simulink model "diff_mobile_model_2"  (R2015b)
settings: Solver=ode5  StartTime=0.0  StopTime=inf  FixedStep=0.01  RelTol=1e-3
values from neighbouring files (symbols this model uses):
  B = 0.1    [param.m]
  I = 0.8    [param.m]
  K = 1    [param.m]
  l = 0.2    [param.m]
  M = 20    [param.m]
  ppr = 1024*5    (= 5120)    [param.m]
  r = 0.065    [param.m]
  T = 0.01    [param.m]
libraries: simulink x2, slctrlblks x1
settings Model: Creator=root  LastModifiedBy=root

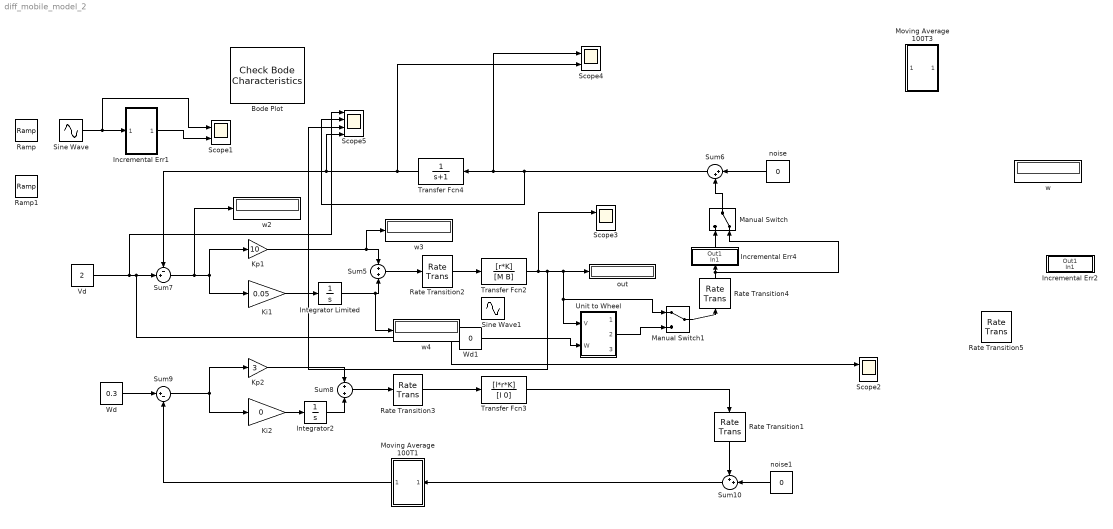
== system diff_mobile_model_2 ==
  Bode Plot : slctrlblks/Model Verification/Check Bode  Characteristics  InstantiateOnLoad=on  SaveOperatingPoints=off  LinearizationIOs={'/Sum7', 1, 'in', 'on', '';'/Transfer Fcn4', 1, 'out', 'on', ''}  LinearizeAt=SnapshotTimes  SnapshotTimes=[0]  TriggerType=rising  SampleTime=0.0001  RateConversionMethod=zoh  PreWarpFreq=10  UseExactDelayModel=off  UseFullBlockNameLabels=off  UseBusSignalLabels=off  enabled=on  stopWhenAssertionFail=off  export=off  ViewDlgPos=[66 1 767 793]  OpenViewOnLoad=on  LaunchViewOnOpen=on  FrequencyUnits=rad/s  MagnitudeUnits=dB  PhaseUnits=deg  TimeUnits=seconds  EnableUpperBound=off  UpperBoundFrequencies=[]  UpperBoundMagnitudes=[]  EnableLowerBound=off  LowerBoundFrequencies=[]  LowerBoundMagnitudes=[]
      settings: SaveToWorkspace=on
  Incremental Err1 : Subsystem
  Incremental Err2 : Subsystem
  Incremental Err4 : Subsystem
  Integrator Limited : Integrator  LimitOutput=on  UpperSaturationLimit=1000  LowerSaturationLimit=-1000
  Integrator2 : Integrator
  Ki1 : Gain  Gain=0.05
  Ki2 : Gain  Gain=0
  Kp1 : Gain  Gain=10
  Kp2 : Gain  Gain=3
  Manual Switch : ManualSwitch  CurrentSetting=0
  Manual Switch1 : ManualSwitch
  Moving Average 100T1 : Subsystem
  Moving Average 100T3 : Subsystem
  Ramp : simulink/Sources/Ramp  slope=1  start=0  X0=0
  Ramp1 : simulink/Sources/Ramp  slope=1  start=0  X0=0
  Rate Transition{1..5} (5 alike) : RateTransition  OutPortSampleTime=control_ts
  Scope{1..4} (4 alike) : Scope  NumInputPorts=2
  Scope5 : Scope  NumInputPorts=4
  Sine Wave : Sin  SampleTime=0
  Sine Wave1 : Sin  SampleTime=0
  Sum10 : Sum  Inputs=++|
  Sum5 : Sum  Inputs=+|+
  Sum6 : Sum  Inputs=|++
  Sum7 : Sum  Inputs=-+|
  Sum8 : Sum  Inputs=+|+
  Sum9 : Sum  Inputs=|+-
  Transfer Fcn2 : TransferFcn  Numerator=[r*K]  Denominator=[M B]
  Transfer Fcn3 : TransferFcn  Numerator=[l*r*K]  Denominator=[I 0]
  Transfer Fcn4 : TransferFcn  Denominator=[1 1]
  Unit to Wheel : Subsystem
  Vd : Constant  Value=2
  Wd : Constant  Value=0.3
  Wd1 : Constant  Value=0
  noise : Constant  Value=0
  noise1 : Constant  Value=0
  out : Display
  w{,2..4} (4 alike) : Display
  wires:
  noise/1 -> Sum6/1
  Kp1/1 -> w3/1, Sum5/1
  Ki1/1 -> Integrator Limited/1
  Sum5/1 -> Rate Transition2/1
  Sum7/1 -> w2/1, Ki1/1, Kp1/1
  Vd/1 -> Scope5/1, Scope2/1, Sum7/2
  Ki2/1 -> Integrator2/1
  Kp2/1 -> Sum8/1
  Integrator2/1 -> Sum8/2
  Sum8/1 -> Rate Transition3/1
  Sum9/1 -> Kp2/1, Ki2/1
  Wd/1 -> Sum9/1
  Transfer Fcn3/1 -> Rate Transition1/1
  noise1/1 -> Sum10/2
  Sum10/1 -> Moving Average 100T1/1(In1)
  Moving Average 100T1/1(Out1) -> Sum9/2
  Sine Wave/1 -> Scope1/1, Incremental Err1/1(In1)
  Incremental Err1/1(Out1) -> Scope1/2
  Rate Transition2/1 -> Transfer Fcn2/1
  Rate Transition1/1 -> Sum10/1
  Rate Transition3/1 -> Transfer Fcn3/1
  Rate Transition4/1 -> Manual Switch/2, Incremental Err4/1(In1)
  Wd1/1 -> Unit to Wheel/2(W)
  Transfer Fcn2/1 -> Scope3/1, Scope5/3, Manual Switch1/1, Unit to Wheel/1(V), out/1
  Manual Switch/1 -> Sum6/2
  Sum6/1 -> Scope5/2, Transfer Fcn4/1, Scope4/1
  Integrator Limited/1 -> w4/1, Sum5/2
  Transfer Fcn4/1 -> Scope4/2, Scope5/4, Sum7/1
  Incremental Err4/1(Out1) -> Manual Switch/1
  Manual Switch1/1 -> Rate Transition4/1
  Unit to Wheel/2(V_enc2) -> Manual Switch1/2

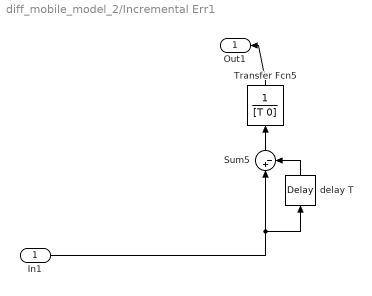
== system diff_mobile_model_2/Incremental Err1 ==
  In1 : Inport
  Sum5 : Sum  Inputs=|+-
  Transfer Fcn5 : TransferFcn  Denominator=[T 0]
  delay T : TransportDelay  DelayTime=T
  Out1 : Outport
  wires:
  Transfer Fcn5/1 -> Out1/1
  delay T/1 -> Sum5/2
  In1/1 -> Sum5/1, delay T/1
  Sum5/1 -> Transfer Fcn5/1

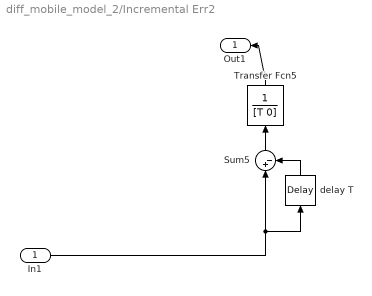
== system diff_mobile_model_2/Incremental Err2 ==
  In1 : Inport
  Sum5 : Sum  Inputs=|+-
  Transfer Fcn5 : TransferFcn  Denominator=[T 0]
  delay T : TransportDelay  DelayTime=T
  Out1 : Outport
  wires:
  Transfer Fcn5/1 -> Out1/1
  delay T/1 -> Sum5/2
  In1/1 -> Sum5/1, delay T/1
  Sum5/1 -> Transfer Fcn5/1

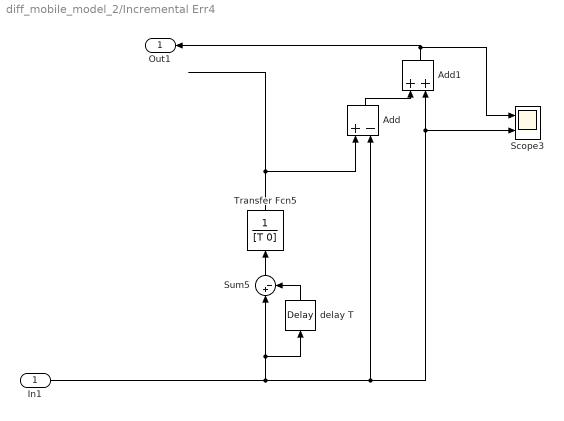
== system diff_mobile_model_2/Incremental Err4 ==
  In1 : Inport
  Add : Sum  Inputs=+-
  Add1 : Sum
  Scope3 : Scope  NumInputPorts=2
  Sum5 : Sum  Inputs=|+-
  Transfer Fcn5 : TransferFcn  Denominator=[T 0]
  delay T : TransportDelay  DelayTime=T
  Out1 : Outport
  wires:
  Transfer Fcn5/1 -> Add/1
  delay T/1 -> Sum5/2
  In1/1 -> Scope3/2, Add1/2, Add/2, Sum5/1, delay T/1
  Sum5/1 -> Transfer Fcn5/1
  Add/1 -> Add1/1
  Add1/1 -> Scope3/1, Out1/1

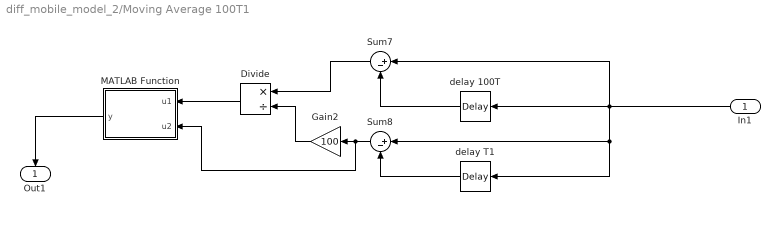
== system diff_mobile_model_2/Moving Average 100T1 ==
  In1 : Inport
  Divide : Product  Inputs=*/
  Gain2 : Gain  Gain=100
  MATLAB Function : MATLAB Function  TreatAsAtomicUnit=on
  Sum7 : Sum  Inputs=|+-
  Sum8 : Sum  Inputs=|+-
  delay 100T : TransportDelay  DelayTime=100
  delay T1 : TransportDelay  DelayTime=T
  Out1 : Outport
  wires:
  Divide/1 -> MATLAB Function/1(u1)
  Sum8/1 -> Gain2/1, MATLAB Function/2(u2)
  delay 100T/1 -> Sum7/2
  delay T1/1 -> Sum8/2
  In1/1 -> delay 100T/1, delay T1/1, Sum8/1, Sum7/1
  MATLAB Function/1(y) -> Out1/1
  Gain2/1 -> Divide/2
  Sum7/1 -> Divide/1

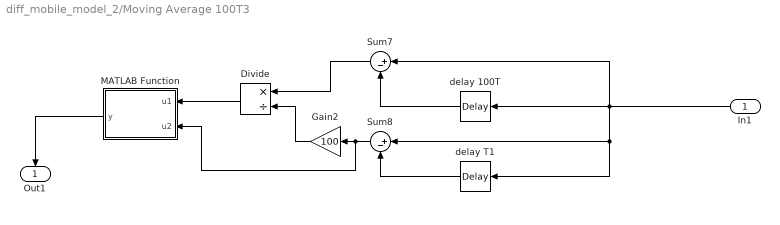
== system diff_mobile_model_2/Moving Average 100T3 ==
  In1 : Inport
  Divide : Product  Inputs=*/
  Gain2 : Gain  Gain=100
  MATLAB Function : MATLAB Function  TreatAsAtomicUnit=on
  Sum7 : Sum  Inputs=|+-
  Sum8 : Sum  Inputs=|+-
  delay 100T : TransportDelay  DelayTime=100
  delay T1 : TransportDelay  DelayTime=T
  Out1 : Outport
  wires:
  Sum7/1 -> Divide/1
  Gain2/1 -> Divide/2
  MATLAB Function/1(y) -> Out1/1
  In1/1 -> Sum7/1, Sum8/1, delay T1/1, delay 100T/1
  delay T1/1 -> Sum8/2
  delay 100T/1 -> Sum7/2
  Sum8/1 -> MATLAB Function/2(u2), Gain2/1
  Divide/1 -> MATLAB Function/1(u1)

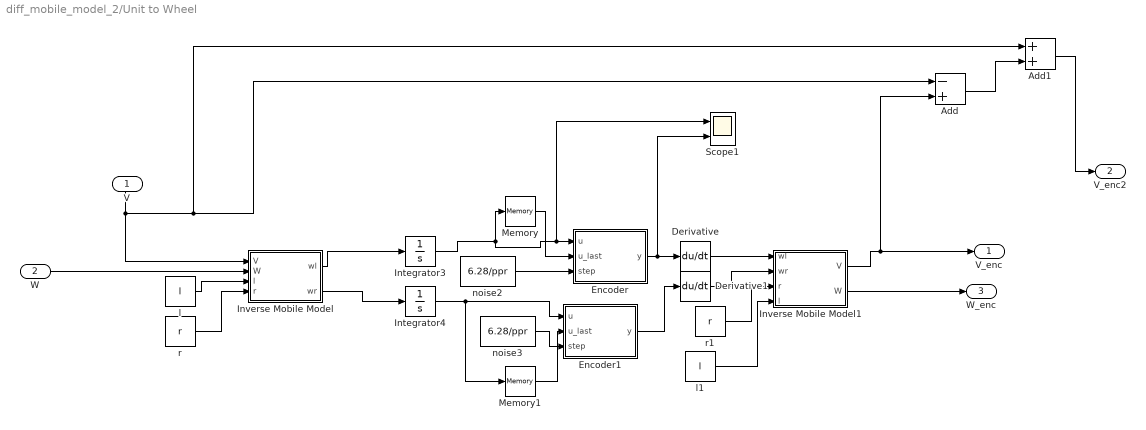
== system diff_mobile_model_2/Unit to Wheel ==
  V : Inport
  W : Inport  Port=2
  Add : Sum  Inputs=-+
  Add1 : Sum
  Derivative : Derivative
  Derivative1 : Derivative
  Encoder : MATLAB Function  TreatAsAtomicUnit=on
  Encoder1 : MATLAB Function  TreatAsAtomicUnit=on
  Integrator3 : Integrator
  Integrator4 : Integrator
  Inverse Mobile Model : MATLAB Function  TreatAsAtomicUnit=on
  Inverse Mobile Model1 : MATLAB Function  TreatAsAtomicUnit=on
  Memory : Memory
  Memory1 : Memory
  Scope1 : Scope  NumInputPorts=2
  l : Constant  Value=l
  l1 : Constant  Value=l
  noise2 : Constant  Value=6.28/ppr
  noise3 : Constant  Value=6.28/ppr
  r : Constant  Value=r
  r1 : Constant  Value=r
  V_enc : Outport
  V_enc2 : Outport  Port=2
  W_enc : Outport  Port=3
  wires:
  Inverse Mobile Model1/1(V) -> Add/2, V_enc/1
  Integrator4/1 -> Memory1/1, Encoder1/1(u)
  Integrator3/1 -> Memory/1, Scope1/1, Encoder/1(u)
  l/1 -> Inverse Mobile Model/3(l)
  Inverse Mobile Model1/2(W) -> W_enc/1
  Inverse Mobile Model/2(wr) -> Integrator4/1
  noise2/1 -> Encoder/3(step)
  W/1 -> Inverse Mobile Model/2(W)
  Inverse Mobile Model/1(wl) -> Integrator3/1
  noise3/1 -> Encoder1/3(step)
  Encoder/1(y) -> Scope1/2, Derivative/1
  V/1 -> Add1/1, Add/1, Inverse Mobile Model/1(V)
  r/1 -> Inverse Mobile Model/4(r)
  Encoder1/1(y) -> Derivative1/1
  r1/1 -> Inverse Mobile Model1/3(r)
  l1/1 -> Inverse Mobile Model1/4(l)
  Derivative/1 -> Inverse Mobile Model1/1(wl)
  Derivative1/1 -> Inverse Mobile Model1/2(wr)
  Memory/1 -> Encoder/2(u_last)
  Memory1/1 -> Encoder1/2(u_last)
  Add/1 -> Add1/2
  Add1/1 -> V_enc2/1

== matlab function diff_mobile_model_2/Moving Average 100T1/MATLAB Function ==
  data: u1 input; y output; u2 input
function y = fcn(u1,u2)
%#codegen

if u2==0
    y=1/100;
else
    y=u1;
end

== matlab function diff_mobile_model_2/Moving Average 100T3/MATLAB Function ==
  data: u1 input; y output; u2 input
function y = fcn(u1,u2)
%#codegen

if u2==0
    y=1/100;
else
    y=u1;
end

== matlab function diff_mobile_model_2/Unit to Wheel/Inverse Mobile Model ==
  data: V input; wl output; W input; wr output; l input; r input
function [wl,wr] = fcn(V,W,l,r)
%#codegen
wl=(2*V-W*2*l)/(2*r);
wr=(2*V+W*2*l)/(2*r);

== matlab function diff_mobile_model_2/Unit to Wheel/Encoder ==
  data: u input; u_last input; y output; step input
function y = fcn(u,u_last,step)
%#codegen
if (u-u_last)>=0
  y=step*floor(u/step);
else
  y=step*ceil(u/step); 
end

== matlab function diff_mobile_model_2/Unit to Wheel/Encoder1 ==
  data: u input; u_last input; y output; step input
function y = fcn(u,u_last,step)
%#codegen
if (u-u_last)>=0
  y=step*floor(u/step);
else
  y=step*ceil(u/step); 
end

== matlab function diff_mobile_model_2/Unit to Wheel/Inverse Mobile Model1 ==
  data: V output; wl input; W output; wr input; r input; l input
function [V,W] = fcn(wl,wr,r,l)
%#codegen
V=r*(wr+wl)/2;
W=r*(wr-wl)/l;
